simulink model "quadcopterModel"  (R2018b)
settings: Solver=ode1  StartTime=0.0  StopTime=param.tfinal  FixedStep=param.dt  RelTol=1e-3
values from neighbouring files (symbols this model uses):
  acc_acom = [1 om_com]    [quadSimRunMain.m]
  acc_bcom = [0 om_com]    [quadSimRunMain.m]
  agyro = 1    [quadSimRunMain.m]
  bgyro = 1    [quadSimRunMain.m]
  gainAcc = 1    [quadSimRunMain.m]
  gainGyro = 1    [quadSimRunMain.m]
  gainPsi = 1    [quadSimRunMain.m]
  gainWind = 1    [quadSimRunMain.m]
  gyro_acom = [1 om_com]    [quadSimRunMain.m]
  gyro_bcom = [1 0]    [quadSimRunMain.m]
  Kdphi = 0.0478*1    (= 0.0478)    [quadSimRunMain.m]
  Kdpsi = 0.067644*1    (= 0.067644)    [quadSimRunMain.m]
  Kdtheta = 0.0478*1    (= 0.0478)    [quadSimRunMain.m]
  Kdx = 15    [quadSimRunMain.m]
  Kdy = 15    [quadSimRunMain.m]
  Kdz = 5.5    [quadSimRunMain.m]
  Kiphi = 0.0098*0    (= 0)    [quadSimRunMain.m]
  Kipsi = 0.045028*.0    (= 0)    [quadSimRunMain.m]
  Kitheta = 0.0098*0    (= 0)    [quadSimRunMain.m]
  Kix = 1    [quadSimRunMain.m]
  Kiy = 1    [quadSimRunMain.m]
  Kiz = 1.5    [quadSimRunMain.m]
  Kpphi = 0.0439*1    (= 0.0439)    [quadSimRunMain.m]
  Kppsi = 0.11038*1    (= 0.11038)    [quadSimRunMain.m]
  Kptheta = 0.0439*1    (= 0.0439)    [quadSimRunMain.m]
  Kpx = 5    [quadSimRunMain.m]
  Kpy = 5    [quadSimRunMain.m]
  Kpz = 3.5    [quadSimRunMain.m]
  Nphi = 1/Tfphi    (= 162.638649449)    [quadSimRunMain.m]
  Npsi = 1/Tfpsi    (= 159.182438993)    [quadSimRunMain.m]
  Ntheta = 1/Tftheta    (= 162.638649449)    [quadSimRunMain.m]
  Nx = 1/0.002099    (= 476.417341591)    [quadSimRunMain.m]
  Ny = 1/0.002099    (= 476.417341591)    [quadSimRunMain.m]
  Nz = 1/0.002099    (= 476.417341591)    [quadSimRunMain.m]
  param = quadparam    [quadDyn.m]    (also in quadDynSimple.m; quadSimRunMain.m; quadcomputeFandT.m; quadcomputeMotorSpeed.m)
  pathSelect = 1    [quadSimRunMain.m]
  windConstant = 1    [quadSimRunMain.m]
  windVarying = 1    [quadSimRunMain.m]
undefined symbols (not defined in the file or in its folder): aHu, aHv, aHw, bHu, bHv, bHw, DiscIntNeverNeededParam
libraries: simulink x7, sharedutil x4
(part 1 of 2)
settings Model: Creator=duho46  LastModifiedBy=duho46

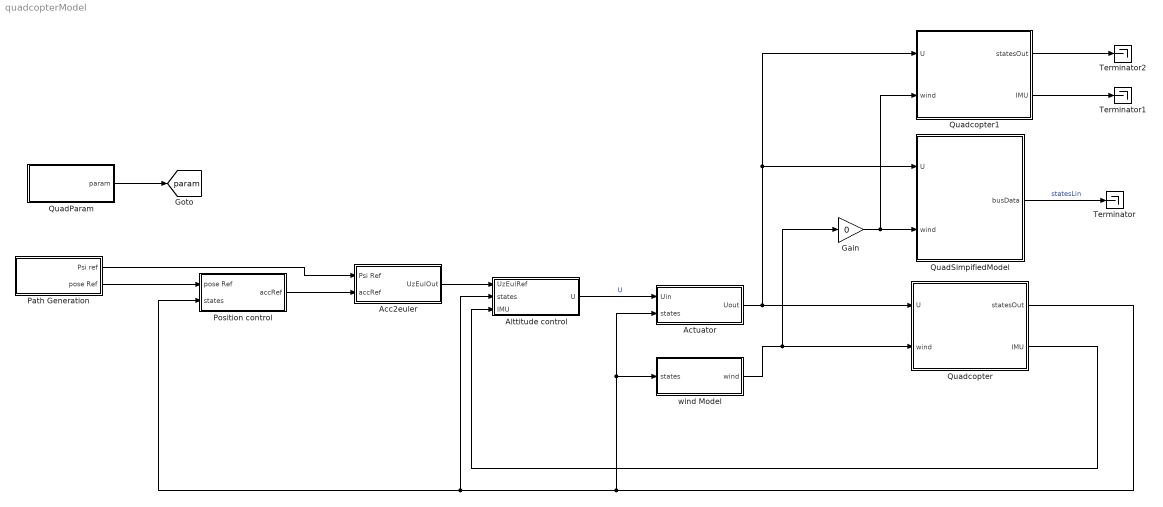
== system quadcopterModel ==
  Acc2euler : Subsystem
  Actuator : Subsystem
  Alttitude control : Subsystem
  Gain : Gain  Gain=0
  Path Generation : Subsystem
  Position control : Subsystem
  QuadParam : Subsystem
  QuadSimpifiedModel : Subsystem
      mask Display: image('C:\Users\duho46\Pictures\DJI Mavic Pro.jpg');
  Quadcopter : Subsystem
  Quadcopter1 : Subsystem
  Terminator : Terminator
  Terminator1 : Terminator
  Terminator2 : Terminator
  wind Model : Subsystem
  tag scope: param=global
  wires:
  Position control/1(accRef) -> Acc2euler/2(accRef)
  Acc2euler/1(UzEulOut) -> Alttitude control/1(UzEulRef)
  Alttitude control/1(U) -> Actuator/1(Uin)  "U"
  Actuator/1(Uout) -> Quadcopter1/1(U), QuadSimpifiedModel/1(U), Quadcopter/1(U)
  Path Generation/2(pose Ref) -> Position control/1(pose Ref)
  Quadcopter/1(statesOut) -> wind Model/1(states), Actuator/2(states), Alttitude control/2(states), Position control/2(states)
  Path Generation/1(Psi ref) -> Acc2euler/1(Psi Ref)
  wind Model/1(wind) -> Gain/1, Quadcopter/2(wind)
  QuadSimpifiedModel/1(busData) -> Terminator/1  "statesLin"
  Quadcopter/2(IMU) -> Alttitude control/3(IMU)
  Gain/1 -> Quadcopter1/2(wind), QuadSimpifiedModel/2(wind)
  QuadParam/1(param) -> [param]
  Quadcopter1/1(statesOut) -> Terminator2/1
  Quadcopter1/2(IMU) -> Terminator1/1

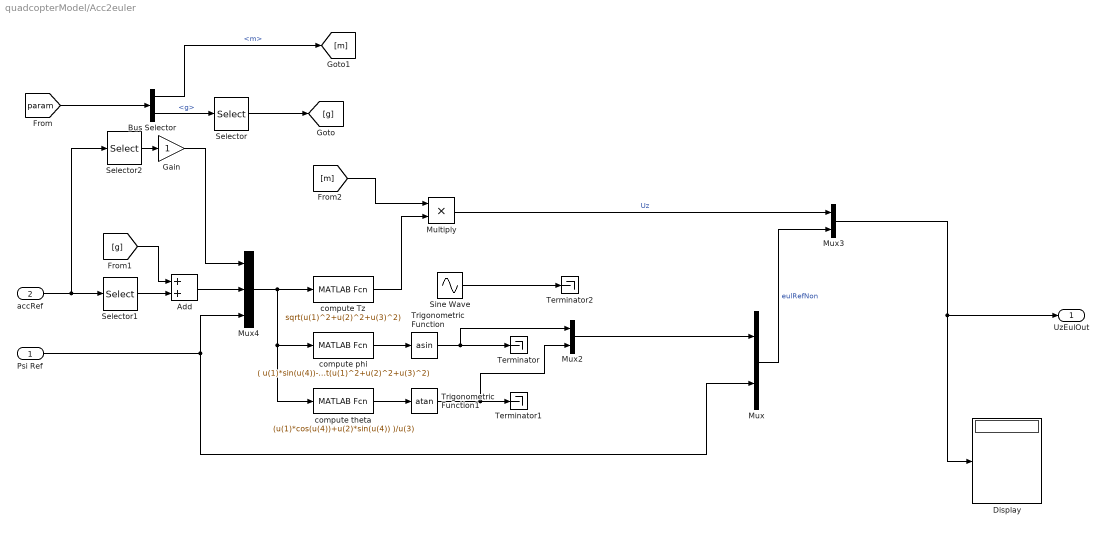
== system quadcopterModel/Acc2euler ==
  Psi Ref : Inport
  accRef : Inport  Port=2
  Add : Sum
  Bus Selector : BusSelector  OutputSignals=m,g
  Display : Display
  Gain : Gain
  Multiply : Product
  Mux : Mux  Inputs=2
  Mux2 : Mux  Inputs=2
  Mux3 : Mux  Inputs=2
  Mux4 : Mux  Inputs=3
  Selector : Selector  InputPortWidth=3  IndexOptions=Index vector (dialog)  Indices=3  OutputSizes=1
  Selector1 : Selector  InputPortWidth=3  IndexOptions=Index vector (dialog)  Indices=3  OutputSizes=1
  Selector2 : Selector  InputPortWidth=3  IndexOptions=Index vector (dialog)  Indices=[1 2]  OutputSizes=1
  Sine Wave : Sin  Amplitude=0.1  Frequency=0.2  SampleTime=0
  Terminator : Terminator
  Terminator1 : Terminator
  Terminator2 : Terminator
  Trigonometric Function : Trigonometry  Operator=asin
  Trigonometric Function1 : Trigonometry  Operator=atan
  compute Tz : MATLABFcn  MATLABFcn=sqrt(u(1)^2+u(2)^2+u(3)^2)  OutputDimensions=1  Output1D=off
  compute phi : MATLABFcn  MATLABFcn=( u(1)*sin(u(4))-u(2)*cos(u(4)) )/sqrt(u(1)^2+u(2)^2+u(3)^2)  OutputDimensions=1  Output1D=off
  compute theta : MATLABFcn  MATLABFcn=(u(1)*cos(u(4))+u(2)*sin(u(4)) )/u(3)  OutputDimensions=1  Output1D=off
  UzEulOut : Outport
  wires:
  [param] -> Bus Selector/1
  Bus Selector/2 -> Selector/1  "<g>"
  Selector/1 -> [g]
  Bus Selector/1 -> [m]  "<m>"
  accRef/1 -> Selector2/1, Selector1/1
  Selector1/1 -> Add/2
  [g] -> Add/1
  Add/1 -> Mux4/2
  [m] -> Multiply/1
  Psi Ref/1 -> Mux/2, Mux4/3
  Multiply/1 -> Mux3/1  "Uz"
  Selector2/1 -> Gain/1
  Mux/1 -> Mux3/2  "eulRefNon"
  Mux4/1 -> compute theta/1, compute phi/1, compute Tz/1
  compute phi/1 -> Trigonometric Function/1
  compute theta/1 -> Trigonometric Function1/1
  Mux3/1 -> Display/1, UzEulOut/1
  Trigonometric Function/1 -> Mux2/1, Terminator/1
  Trigonometric Function1/1 -> Mux2/2, Terminator1/1
  Gain/1 -> Mux4/1
  Mux2/1 -> Mux/1
  Sine Wave/1 -> Terminator2/1
  compute Tz/1 -> Multiply/2

== system quadcopterModel/Actuator ==
  Uin : Inport
  states : Inport  Port=2
  Bus Selector : BusSelector  OutputSignals=T,invT
  Constant : Constant  Value=diag([1 1 1 1])
  Display : Display
  Display1 : Display
  Multiply : Product  Multiplication=Matrix(*)
  Multiply1 : Product  Inputs=3  Multiplication=Matrix(*)
  Mux : Mux  Inputs=2
  Saturation1 : Saturate  UpperLimit=60000  LowerLimit=0
  Scope : Scope
  Scope1 : Scope
  Terminator : Terminator
  Uout : Outport
  wires:
  Uin/1 -> Mux/2, Display/1, Multiply/2
  states/1 -> Terminator/1
  [param] -> Bus Selector/1
  Multiply/1 -> Saturation1/1  "omRotor2"
  Multiply1/1 -> Mux/1, Display1/1, Uout/1
  Constant/1 -> Multiply1/1
  Bus Selector/2 -> Multiply/1  "<invT>"
  Bus Selector/1 -> Multiply1/2  "<T>"
  Mux/1 -> Scope/1
  Saturation1/1 -> Scope1/1, Multiply1/3

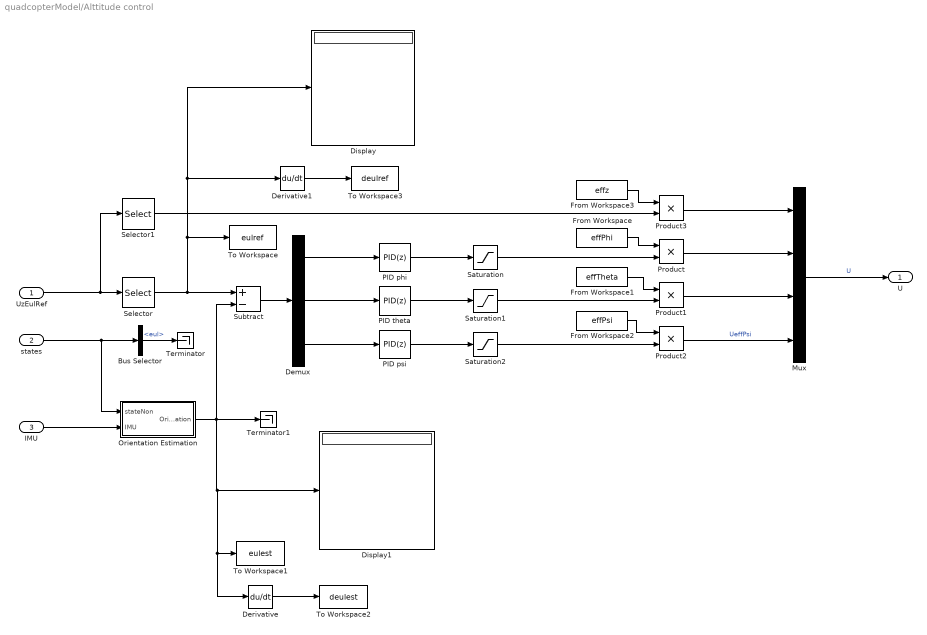
== system quadcopterModel/Alttitude control ==
  UzEulRef : Inport
  states : Inport  Port=2
  IMU : Inport  Port=3
  Bus Selector : BusSelector  OutputSignals=eul
  Demux : Demux  Outputs=3
  Derivative : Derivative
  Derivative1 : Derivative
  Display : Display
  Display1 : Display
  From Workspace : FromWorkspace  VariableName=effPhi  SampleTime=0
  From Workspace1 : FromWorkspace  VariableName=effTheta  SampleTime=0
  From Workspace2 : FromWorkspace  VariableName=effPsi  SampleTime=0
  From Workspace3 : FromWorkspace  VariableName=effz  SampleTime=0
  Mux : Mux
  Orientation Estimation : Subsystem
  PID phi : simulink/Continuous/PID Controller  Controller=PID  Form=Parallel  TimeDomain=Discrete-time  SampleTime=-1  IntegratorMethod=Forward Euler  FilterMethod=Forward Euler  ControllerParametersSource=internal  P=Kpphi  I=Kiphi*0  D=Kdphi  UseFilter=off  N=Nphi  TunerSelectOption=Transfer Function Based (PID Tuner App)  InitialConditionSource=internal  InitialConditionForIntegrator=0  InitialConditionForFilter=0  DifferentiatorICPrevScaledInput=0  ExternalReset=none  TrackingMode=off  Kt=1  LimitOutput=off  UpperSaturationLimit=inf  LowerSaturationLimit=-inf  LinearizeAsGain=on  AntiWindupMode=none  Kb=1  POutMin=[]  POutMax=[]  IOutMin=[]  IOutMax=[]  DOutMin=[]  DOutMax=[]  NOutMin=[]  NOutMax=[]  SumOutMin=[]  SumOutMax=[]  SaturationOutMin=[]  SaturationOutMax=[]  PParamMin=[]  PParamMax=[]  IParamMin=[]  IParamMax=[]  DParamMin=[]  DParamMax=[]  NParamMin=[]  NParamMax=[]  KbParamMin=[]  KbParamMax=[]  KtParamMin=[]  KtParamMax=[]  KbOutMin=[]  KbOutMax=[]  KtOutMin=[]  KtOutMax=[]  IntegratorOutMin=[]  IntegratorOutMax=[]  FilterOutMin=[]  FilterOutMax=[]  SumI1OutMin=[]  SumI1OutMax=[]  SumI2OutMin=[]  SumI2OutMax=[]  SumI3OutMin=[]  SumI3OutMax=[]  SumI4OutMin=[]  SumI4OutMax=[]  SumDOutMin=[]  SumDOutMax=[]  DifferentiatorOutMin=[]  DifferentiatorOutMax=[]  FilterDiffOutCoefMin=[]  FilterDiffOutCoefMax=[]  ReciprocalOutMin=[]  ReciprocalOutMax=[]  SumDenOutMin=[]  SumDenOutMax=[]  SumNumOutMin=[]  SumNumOutMax=[]  DivideOutMin=[]  DivideOutMax=[]  IntegratorContinuousStateAttributes=''  IntegratorStateMustResolveToSignalObject=off  IntegratorRTWStateStorageClass=Auto  FilterContinuousStateAttributes=''  FilterStateMustResolveToSignalObject=off  FilterRTWStateStorageClass=Auto  ParallelPVariant=InternalParameters  IdealPVariant=Disabled  IVariant=InternalParameters  DVariant=InternalParameters  IntegratorVariant=Discrete  SatVariant=Disabled  AWVariant=Passthrough  PCopyVariant=Disabled  TRVariant=Disabled  FdbkBlocksVariant=Forward  IdealPFdbkVariant=Disabled  SatFdbkVariant=Disabled  DerivativeFilterVariant=Differentiator  NVariant=Passthrough  NCopyVariant=Disabled_SignalSpec  FilterICVariant=InternalICsDifferentiator  IntegratorICVariant=InternalICs  ExternalResetVariant=Disabled  TRSumVariant=Passthrough  SumFdbkVariant=Disabled  SumVariant=Sum_PID
  PID psi : simulink/Continuous/PID Controller  Controller=PID  Form=Parallel  TimeDomain=Discrete-time  SampleTime=-1  IntegratorMethod=Forward Euler  FilterMethod=Forward Euler  ControllerParametersSource=internal  P=Kppsi  I=Kipsi  D=Kdpsi  UseFilter=off  N=Npsi  TunerSelectOption=Transfer Function Based (PID Tuner App)  InitialConditionSource=internal  InitialConditionForIntegrator=0  InitialConditionForFilter=0  DifferentiatorICPrevScaledInput=0  ExternalReset=none  TrackingMode=off  Kt=1  LimitOutput=off  UpperSaturationLimit=inf  LowerSaturationLimit=-inf  LinearizeAsGain=on  AntiWindupMode=none  Kb=1  POutMin=[]  POutMax=[]  IOutMin=[]  IOutMax=[]  DOutMin=[]  DOutMax=[]  NOutMin=[]  NOutMax=[]  SumOutMin=[]  SumOutMax=[]  SaturationOutMin=[]  SaturationOutMax=[]  PParamMin=[]  PParamMax=[]  IParamMin=[]  IParamMax=[]  DParamMin=[]  DParamMax=[]  NParamMin=[]  NParamMax=[]  KbParamMin=[]  KbParamMax=[]  KtParamMin=[]  KtParamMax=[]  KbOutMin=[]  KbOutMax=[]  KtOutMin=[]  KtOutMax=[]  IntegratorOutMin=[]  IntegratorOutMax=[]  FilterOutMin=[]  FilterOutMax=[]  SumI1OutMin=[]  SumI1OutMax=[]  SumI2OutMin=[]  SumI2OutMax=[]  SumI3OutMin=[]  SumI3OutMax=[]  SumI4OutMin=[]  SumI4OutMax=[]  SumDOutMin=[]  SumDOutMax=[]  DifferentiatorOutMin=[]  DifferentiatorOutMax=[]  FilterDiffOutCoefMin=[]  FilterDiffOutCoefMax=[]  ReciprocalOutMin=[]  ReciprocalOutMax=[]  SumDenOutMin=[]  SumDenOutMax=[]  SumNumOutMin=[]  SumNumOutMax=[]  DivideOutMin=[]  DivideOutMax=[]  IntegratorContinuousStateAttributes=''  IntegratorStateMustResolveToSignalObject=off  IntegratorRTWStateStorageClass=Auto  FilterContinuousStateAttributes=''  FilterStateMustResolveToSignalObject=off  FilterRTWStateStorageClass=Auto  ParallelPVariant=InternalParameters  IdealPVariant=Disabled  IVariant=InternalParameters  DVariant=InternalParameters  IntegratorVariant=Discrete  SatVariant=Disabled  AWVariant=Passthrough  PCopyVariant=Disabled  TRVariant=Disabled  FdbkBlocksVariant=Forward  IdealPFdbkVariant=Disabled  SatFdbkVariant=Disabled  DerivativeFilterVariant=Differentiator  NVariant=Passthrough  NCopyVariant=Disabled_SignalSpec  FilterICVariant=InternalICsDifferentiator  IntegratorICVariant=InternalICs  ExternalResetVariant=Disabled  TRSumVariant=Passthrough  SumFdbkVariant=Disabled  SumVariant=Sum_PID
  PID theta : simulink/Continuous/PID Controller  Controller=PID  Form=Parallel  TimeDomain=Discrete-time  SampleTime=-1  IntegratorMethod=Forward Euler  FilterMethod=Forward Euler  ControllerParametersSource=internal  P=Kptheta  I=Kitheta*0  D=Kdtheta  UseFilter=off  N=Ntheta  TunerSelectOption=Transfer Function Based (PID Tuner App)  InitialConditionSource=internal  InitialConditionForIntegrator=0  InitialConditionForFilter=0  DifferentiatorICPrevScaledInput=0  ExternalReset=none  TrackingMode=off  Kt=1  LimitOutput=off  UpperSaturationLimit=inf  LowerSaturationLimit=-inf  LinearizeAsGain=on  AntiWindupMode=none  Kb=1  POutMin=[]  POutMax=[]  IOutMin=[]  IOutMax=[]  DOutMin=[]  DOutMax=[]  NOutMin=[]  NOutMax=[]  SumOutMin=[]  SumOutMax=[]  SaturationOutMin=[]  SaturationOutMax=[]  PParamMin=[]  PParamMax=[]  IParamMin=[]  IParamMax=[]  DParamMin=[]  DParamMax=[]  NParamMin=[]  NParamMax=[]  KbParamMin=[]  KbParamMax=[]  KtParamMin=[]  KtParamMax=[]  KbOutMin=[]  KbOutMax=[]  KtOutMin=[]  KtOutMax=[]  IntegratorOutMin=[]  IntegratorOutMax=[]  FilterOutMin=[]  FilterOutMax=[]  SumI1OutMin=[]  SumI1OutMax=[]  SumI2OutMin=[]  SumI2OutMax=[]  SumI3OutMin=[]  SumI3OutMax=[]  SumI4OutMin=[]  SumI4OutMax=[]  SumDOutMin=[]  SumDOutMax=[]  DifferentiatorOutMin=[]  DifferentiatorOutMax=[]  FilterDiffOutCoefMin=[]  FilterDiffOutCoefMax=[]  ReciprocalOutMin=[]  ReciprocalOutMax=[]  SumDenOutMin=[]  SumDenOutMax=[]  SumNumOutMin=[]  SumNumOutMax=[]  DivideOutMin=[]  DivideOutMax=[]  IntegratorContinuousStateAttributes=''  IntegratorStateMustResolveToSignalObject=off  IntegratorRTWStateStorageClass=Auto  FilterContinuousStateAttributes=''  FilterStateMustResolveToSignalObject=off  FilterRTWStateStorageClass=Auto  ParallelPVariant=InternalParameters  IdealPVariant=Disabled  IVariant=InternalParameters  DVariant=InternalParameters  IntegratorVariant=Discrete  SatVariant=Disabled  AWVariant=Passthrough  PCopyVariant=Disabled  TRVariant=Disabled  FdbkBlocksVariant=Forward  IdealPFdbkVariant=Disabled  SatFdbkVariant=Disabled  DerivativeFilterVariant=Differentiator  NVariant=Passthrough  NCopyVariant=Disabled_SignalSpec  FilterICVariant=InternalICsDifferentiator  IntegratorICVariant=InternalICs  ExternalResetVariant=Disabled  TRSumVariant=Passthrough  SumFdbkVariant=Disabled  SumVariant=Sum_PID
  Product{,1..3} (4 alike) : Product
  Saturation : Saturate  UpperLimit=1  LowerLimit=-1
  Saturation1 : Saturate  UpperLimit=1  LowerLimit=-1
  Saturation2 : Saturate  UpperLimit=10  LowerLimit=-10
  Selector : Selector  InputPortWidth=4  IndexOptions=Index vector (dialog)  Indices=[2 3 4]  OutputSizes=1
  Selector1 : Selector  InputPortWidth=4  IndexOptions=Index vector (dialog)  Indices=1  OutputSizes=1
  Subtract : Sum  Inputs=+-
  Terminator : Terminator
  Terminator1 : Terminator
  To Workspace : ToWorkspace  VariableName=eulref  SampleTime=-1
  To Workspace1 : ToWorkspace  VariableName=eulest  SampleTime=-1
  To Workspace2 : ToWorkspace  VariableName=deulest  SampleTime=-1
  To Workspace3 : ToWorkspace  VariableName=deulref  SampleTime=-1
  U : Outport
  wires:
  states/1 -> Orientation Estimation/1(stateNon), Bus Selector/1
  UzEulRef/1 -> Selector1/1, Selector/1
  Product3/1 -> Mux/1
  From Workspace3/1 -> Product3/1
  Demux/1 -> PID phi/1
  From Workspace2/1 -> Product2/1
  Product2/1 -> Mux/4  "UeffPsi"
  Mux/1 -> U/1  "U"
  Selector1/1 -> Product3/2
  PID psi/1 -> Saturation2/1
  Product1/1 -> Mux/3
  From Workspace1/1 -> Product1/1
  Demux/3 -> PID psi/1
  PID theta/1 -> Saturation1/1
  Product/1 -> Mux/2
  PID phi/1 -> Saturation/1
  Demux/2 -> PID theta/1
  From Workspace/1 -> Product/1
  Subtract/1 -> Demux/1
  Selector/1 -> To Workspace/1, Derivative1/1, Display/1, Subtract/1
  IMU/1 -> Orientation Estimation/2(IMU)
  Bus Selector/1 -> Terminator/1  "<eul>"
  Orientation Estimation/1(Orientation) -> Subtract/2, Derivative/1, To Workspace1/1, Display1/1, Terminator1/1
  Saturation/1 -> Product/2
  Saturation1/1 -> Product1/2
  Saturation2/1 -> Product2/2
  Derivative/1 -> To Workspace2/1
  Derivative1/1 -> To Workspace3/1

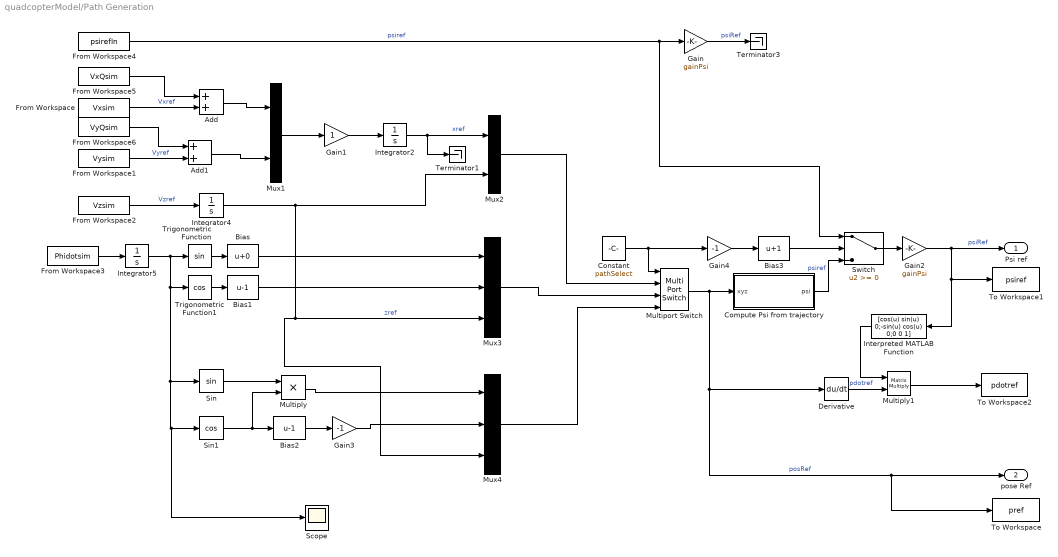
== system quadcopterModel/Path Generation ==
  Add : Sum
  Add1 : Sum
  Bias : Bias
  Bias1 : Bias  Bias=-1
  Bias2 : Bias  Bias=-1
  Bias3 : Bias  Bias=1
  Compute Psi from trajectory : Subsystem
  Constant : Constant  Value=pathSelect
  Derivative : Derivative
  From Workspace : FromWorkspace  VariableName=Vxsim  SampleTime=0
  From Workspace1 : FromWorkspace  VariableName=Vysim  SampleTime=0
  From Workspace2 : FromWorkspace  VariableName=Vzsim  SampleTime=0
  From Workspace3 : FromWorkspace  VariableName=Phidotsim  SampleTime=0
  From Workspace4 : FromWorkspace  VariableName=psirefIn  SampleTime=0
  From Workspace5 : FromWorkspace  VariableName=VxQsim  SampleTime=0
  From Workspace6 : FromWorkspace  VariableName=VyQsim  SampleTime=0
  Gain : Gain  Gain=gainPsi
  Gain1 : Gain
  Gain2 : Gain  Gain=gainPsi
  Gain3 : Gain  Gain=-1
  Gain4 : Gain  Gain=-1
  Integrator2 : Integrator
  Integrator4 : Integrator  InitialCondition=8
  Integrator5 : Integrator
  Interpreted MATLAB Function : MATLABFcn  MATLABFcn=[cos(u) sin(u) 0;-sin(u) cos(u) 0;0 0 1]  OutputDimensions=[3 3]  Output1D=off
  Multiply : Product
  Multiply1 : Product  Multiplication=Matrix(*)
  Multiport Switch : MultiPortSwitch
  Mux1 : Mux  Inputs=2
  Mux2 : Mux  Inputs=2
  Mux3 : Mux  Inputs=3
  Mux4 : Mux  Inputs=3
  Scope : Scope
  Sin : Trigonometry
  Sin1 : Trigonometry  Operator=cos
  Switch : Switch
  Terminator1 : Terminator
  Terminator3 : Terminator
  To Workspace : ToWorkspace  VariableName=pref  SampleTime=-1
  To Workspace1 : ToWorkspace  VariableName=psiref  SampleTime=-1
  To Workspace2 : ToWorkspace  VariableName=pdotref  SampleTime=-1
  Trigonometric Function : Trigonometry
  Trigonometric Function1 : Trigonometry  Operator=cos
  Psi ref : Outport
  pose Ref : Outport  Port=2
  wires:
  Mux1/1 -> Gain1/1
  From Workspace4/1 -> Switch/1, Gain/1  "psiref"
  Bias1/1 -> Mux3/2
  Bias/1 -> Mux3/1
  Trigonometric Function/1 -> Bias/1
  Trigonometric Function1/1 -> Bias1/1
  From Workspace3/1 -> Integrator5/1
  Integrator5/1 -> Trigonometric Function/1, Scope/1, Sin1/1, Sin/1, Trigonometric Function1/1
  From Workspace2/1 -> Integrator4/1  "Vzref"
  Integrator4/1 -> Mux2/2, Mux4/3, Mux3/3  "zref"
  Gain1/1 -> Integrator2/1
  Integrator2/1 -> Mux2/1, Terminator1/1  "xref"
  Sin1/1 -> Bias2/1, Multiply/2
  Sin/1 -> Multiply/1
  Multiport Switch/1 -> Compute Psi from trajectory/1(xyz), Derivative/1, To Workspace/1, pose Ref/1  "posRef"
  Gain/1 -> Terminator3/1  "psiRef"
  Bias2/1 -> Gain3/1
  Gain2/1 -> Psi ref/1, To Workspace1/1, Interpreted MATLAB Function/1  "psiRef"
  Mux2/1 -> Multiport Switch/2
  Mux3/1 -> Multiport Switch/3
  Mux4/1 -> Multiport Switch/4
  Constant/1 -> Multiport Switch/1, Gain4/1
  Multiply/1 -> Mux4/1
  Gain3/1 -> Mux4/2
  Compute Psi from trajectory/1(psi) -> Switch/3  "psiref"
  Switch/1 -> Gain2/1
  Gain4/1 -> Bias3/1
  Bias3/1 -> Switch/2
  Interpreted MATLAB Function/1 -> Multiply1/1
  Derivative/1 -> Multiply1/2  "pdotref"
  Multiply1/1 -> To Workspace2/1
  From Workspace/1 -> Add/2  "Vxref"
  From Workspace1/1 -> Add1/2  "Vyref"
  From Workspace6/1 -> Add1/1
  Add1/1 -> Mux1/2
  Add/1 -> Mux1/1
  From Workspace5/1 -> Add/1

== system quadcopterModel/Position control ==
  pose Ref : Inport
  states : Inport  Port=2
  Bus Selector : BusSelector  OutputSignals=p
  Demux : Demux  Outputs=3
  Demux1 : Demux  Outputs=3
  Mux : Mux  Inputs=3
  PID x : simulink/Continuous/PID Controller  Controller=PID  Form=Parallel  TimeDomain=Discrete-time  SampleTime=-1  IntegratorMethod=Forward Euler  FilterMethod=Forward Euler  ControllerParametersSource=internal  P=Kpx  I=Kix  D=Kdx  UseFilter=off  N=Nx  TunerSelectOption=Transfer Function Based (PID Tuner App)  InitialConditionSource=internal  InitialConditionForIntegrator=0  InitialConditionForFilter=0  DifferentiatorICPrevScaledInput=0  ExternalReset=none  TrackingMode=off  Kt=1  LimitOutput=off  UpperSaturationLimit=inf  LowerSaturationLimit=-inf  LinearizeAsGain=on  AntiWindupMode=none  Kb=1  POutMin=[]  POutMax=[]  IOutMin=[]  IOutMax=[]  DOutMin=[]  DOutMax=[]  NOutMin=[]  NOutMax=[]  SumOutMin=[]  SumOutMax=[]  SaturationOutMin=[]  SaturationOutMax=[]  PParamMin=[]  PParamMax=[]  IParamMin=[]  IParamMax=[]  DParamMin=[]  DParamMax=[]  NParamMin=[]  NParamMax=[]  KbParamMin=[]  KbParamMax=[]  KtParamMin=[]  KtParamMax=[]  KbOutMin=[]  KbOutMax=[]  KtOutMin=[]  KtOutMax=[]  IntegratorOutMin=[]  IntegratorOutMax=[]  FilterOutMin=[]  FilterOutMax=[]  SumI1OutMin=[]  SumI1OutMax=[]  SumI2OutMin=[]  SumI2OutMax=[]  SumI3OutMin=[]  SumI3OutMax=[]  SumI4OutMin=[]  SumI4OutMax=[]  SumDOutMin=[]  SumDOutMax=[]  DifferentiatorOutMin=[]  DifferentiatorOutMax=[]  FilterDiffOutCoefMin=[]  FilterDiffOutCoefMax=[]  ReciprocalOutMin=[]  ReciprocalOutMax=[]  SumDenOutMin=[]  SumDenOutMax=[]  SumNumOutMin=[]  SumNumOutMax=[]  DivideOutMin=[]  DivideOutMax=[]  IntegratorContinuousStateAttributes=''  IntegratorStateMustResolveToSignalObject=off  IntegratorRTWStateStorageClass=Auto  FilterContinuousStateAttributes=''  FilterStateMustResolveToSignalObject=off  FilterRTWStateStorageClass=Auto  ParallelPVariant=InternalParameters  IdealPVariant=Disabled  IVariant=InternalParameters  DVariant=InternalParameters  IntegratorVariant=Discrete  SatVariant=Disabled  AWVariant=Passthrough  PCopyVariant=Disabled  TRVariant=Disabled  FdbkBlocksVariant=Forward  IdealPFdbkVariant=Disabled  SatFdbkVariant=Disabled  DerivativeFilterVariant=Differentiator  NVariant=Passthrough  NCopyVariant=Disabled_SignalSpec  FilterICVariant=InternalICsDifferentiator  IntegratorICVariant=InternalICs  ExternalResetVariant=Disabled  TRSumVariant=Passthrough  SumFdbkVariant=Disabled  SumVariant=Sum_PID
  PID y : simulink/Continuous/PID Controller  Controller=PID  Form=Parallel  TimeDomain=Discrete-time  SampleTime=-1  IntegratorMethod=Forward Euler  FilterMethod=Forward Euler  ControllerParametersSource=internal  P=Kpy  I=Kiy  D=Kdy  UseFilter=off  N=Ny  TunerSelectOption=Transfer Function Based (PID Tuner App)  InitialConditionSource=internal  InitialConditionForIntegrator=0  InitialConditionForFilter=0  DifferentiatorICPrevScaledInput=0  ExternalReset=none  TrackingMode=off  Kt=1  LimitOutput=off  UpperSaturationLimit=inf  LowerSaturationLimit=-inf  LinearizeAsGain=on  AntiWindupMode=none  Kb=1  POutMin=[]  POutMax=[]  IOutMin=[]  IOutMax=[]  DOutMin=[]  DOutMax=[]  NOutMin=[]  NOutMax=[]  SumOutMin=[]  SumOutMax=[]  SaturationOutMin=[]  SaturationOutMax=[]  PParamMin=[]  PParamMax=[]  IParamMin=[]  IParamMax=[]  DParamMin=[]  DParamMax=[]  NParamMin=[]  NParamMax=[]  KbParamMin=[]  KbParamMax=[]  KtParamMin=[]  KtParamMax=[]  KbOutMin=[]  KbOutMax=[]  KtOutMin=[]  KtOutMax=[]  IntegratorOutMin=[]  IntegratorOutMax=[]  FilterOutMin=[]  FilterOutMax=[]  SumI1OutMin=[]  SumI1OutMax=[]  SumI2OutMin=[]  SumI2OutMax=[]  SumI3OutMin=[]  SumI3OutMax=[]  SumI4OutMin=[]  SumI4OutMax=[]  SumDOutMin=[]  SumDOutMax=[]  DifferentiatorOutMin=[]  DifferentiatorOutMax=[]  FilterDiffOutCoefMin=[]  FilterDiffOutCoefMax=[]  ReciprocalOutMin=[]  ReciprocalOutMax=[]  SumDenOutMin=[]  SumDenOutMax=[]  SumNumOutMin=[]  SumNumOutMax=[]  DivideOutMin=[]  DivideOutMax=[]  IntegratorContinuousStateAttributes=''  IntegratorStateMustResolveToSignalObject=off  IntegratorRTWStateStorageClass=Auto  FilterContinuousStateAttributes=''  FilterStateMustResolveToSignalObject=off  FilterRTWStateStorageClass=Auto  ParallelPVariant=InternalParameters  IdealPVariant=Disabled  IVariant=InternalParameters  DVariant=InternalParameters  IntegratorVariant=Discrete  SatVariant=Disabled  AWVariant=Passthrough  PCopyVariant=Disabled  TRVariant=Disabled  FdbkBlocksVariant=Forward  IdealPFdbkVariant=Disabled  SatFdbkVariant=Disabled  DerivativeFilterVariant=Differentiator  NVariant=Passthrough  NCopyVariant=Disabled_SignalSpec  FilterICVariant=InternalICsDifferentiator  IntegratorICVariant=InternalICs  ExternalResetVariant=Disabled  TRSumVariant=Passthrough  SumFdbkVariant=Disabled  SumVariant=Sum_PID
  PID z : simulink/Continuous/PID Controller  Controller=PID  Form=Parallel  TimeDomain=Discrete-time  SampleTime=-1  IntegratorMethod=Forward Euler  FilterMethod=Forward Euler  ControllerParametersSource=internal  P=Kpz  I=Kiz  D=Kdz  UseFilter=off  N=Nz  TunerSelectOption=Transfer Function Based (PID Tuner App)  InitialConditionSource=internal  InitialConditionForIntegrator=0  InitialConditionForFilter=0  DifferentiatorICPrevScaledInput=0  ExternalReset=none  TrackingMode=off  Kt=1  LimitOutput=off  UpperSaturationLimit=inf  LowerSaturationLimit=-inf  LinearizeAsGain=on  AntiWindupMode=none  Kb=1  POutMin=[]  POutMax=[]  IOutMin=[]  IOutMax=[]  DOutMin=[]  DOutMax=[]  NOutMin=[]  NOutMax=[]  SumOutMin=[]  SumOutMax=[]  SaturationOutMin=[]  SaturationOutMax=[]  PParamMin=[]  PParamMax=[]  IParamMin=[]  IParamMax=[]  DParamMin=[]  DParamMax=[]  NParamMin=[]  NParamMax=[]  KbParamMin=[]  KbParamMax=[]  KtParamMin=[]  KtParamMax=[]  KbOutMin=[]  KbOutMax=[]  KtOutMin=[]  KtOutMax=[]  IntegratorOutMin=[]  IntegratorOutMax=[]  FilterOutMin=[]  FilterOutMax=[]  SumI1OutMin=[]  SumI1OutMax=[]  SumI2OutMin=[]  SumI2OutMax=[]  SumI3OutMin=[]  SumI3OutMax=[]  SumI4OutMin=[]  SumI4OutMax=[]  SumDOutMin=[]  SumDOutMax=[]  DifferentiatorOutMin=[]  DifferentiatorOutMax=[]  FilterDiffOutCoefMin=[]  FilterDiffOutCoefMax=[]  ReciprocalOutMin=[]  ReciprocalOutMax=[]  SumDenOutMin=[]  SumDenOutMax=[]  SumNumOutMin=[]  SumNumOutMax=[]  DivideOutMin=[]  DivideOutMax=[]  IntegratorContinuousStateAttributes=''  IntegratorStateMustResolveToSignalObject=off  IntegratorRTWStateStorageClass=Auto  FilterContinuousStateAttributes=''  FilterStateMustResolveToSignalObject=off  FilterRTWStateStorageClass=Auto  ParallelPVariant=InternalParameters  IdealPVariant=Disabled  IVariant=InternalParameters  DVariant=InternalParameters  IntegratorVariant=Discrete  SatVariant=Disabled  AWVariant=Passthrough  PCopyVariant=Disabled  TRVariant=Disabled  FdbkBlocksVariant=Forward  IdealPFdbkVariant=Disabled  SatFdbkVariant=Disabled  DerivativeFilterVariant=Differentiator  NVariant=Passthrough  NCopyVariant=Disabled_SignalSpec  FilterICVariant=InternalICsDifferentiator  IntegratorICVariant=InternalICs  ExternalResetVariant=Disabled  TRSumVariant=Passthrough  SumFdbkVariant=Disabled  SumVariant=Sum_PID
  Scope : Scope
  Scope1 : Scope
  Sum : Sum  Inputs=|+-
  Terminator : Terminator
  To Workspace : ToWorkspace  VariableName=accRef  SampleTime=-1
  accRef : Outport
  wires:
  Sum/1 -> Demux1/1, Demux/1
  Demux/2 -> PID y/1
  Demux/1 -> PID x/1
  pose Ref/1 -> Sum/1
  Mux/1 -> To Workspace/1, accRef/1  "accRef"
  PID z/1 -> Mux/3
  PID y/1 -> Mux/2
  PID x/1 -> Mux/1
  Demux/3 -> PID z/1
  states/1 -> Bus Selector/1
  Bus Selector/1 -> Sum/2  "<p>"
  Demux1/1 -> Scope/1
  Demux1/2 -> Scope1/1
  Demux1/3 -> Terminator/1

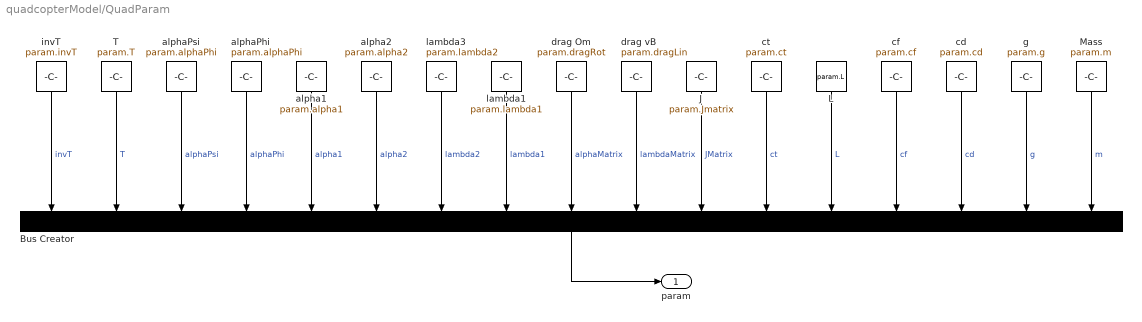
== system quadcopterModel/QuadParam ==
  Bus Creator : BusCreator  Inputs=17
  J : Constant  Value=param.Jmatrix  VectorParams1D=off  OutDataTypeStr=double  SampleTime=-1
  L : Constant  Value=param.L
  Mass : Constant  Value=param.m
  T : Constant  Value=param.T
  "alpha1 " : Constant  Value=param.alpha1
  alpha2 : Constant  Value=param.alpha2
  alphaPhi : Constant  Value=param.alphaPhi
  alphaPsi : Constant  Value=param.alphaPhi
  cd : Constant  Value=param.cd
  cf : Constant  Value=param.cf
  ct : Constant  Value=param.ct
  drag Om : Constant  Value=param.dragRot  VectorParams1D=off
  drag vB : Constant  Value=param.dragLin  VectorParams1D=off
  g : Constant  Value=param.g
  invT : Constant  Value=param.invT
  lambda1 : Constant  Value=param.lambda1
  lambda3 : Constant  Value=param.lambda2
  param : Outport
  wires:
  invT/1 -> Bus Creator/1  "invT"
  T/1 -> Bus Creator/2  "T"
  alphaPsi/1 -> Bus Creator/3  "alphaPsi"
  alphaPhi/1 -> Bus Creator/4  "alphaPhi"
  "alpha1 "/1 -> Bus Creator/5  "alpha1"
  alpha2/1 -> Bus Creator/6  "alpha2"
  lambda3/1 -> Bus Creator/7  "lambda2"
  lambda1/1 -> Bus Creator/8  "lambda1"
  drag Om/1 -> Bus Creator/9  "alphaMatrix"
  drag vB/1 -> Bus Creator/10  "lambdaMatrix"
  J/1 -> Bus Creator/11  "JMatrix"
  ct/1 -> Bus Creator/12  "ct"
  L/1 -> Bus Creator/13  "L"
  cf/1 -> Bus Creator/14  "cf"
  cd/1 -> Bus Creator/15  "cd"
  g/1 -> Bus Creator/16  "g"
  Mass/1 -> Bus Creator/17  "m"
  Bus Creator/1 -> param/1

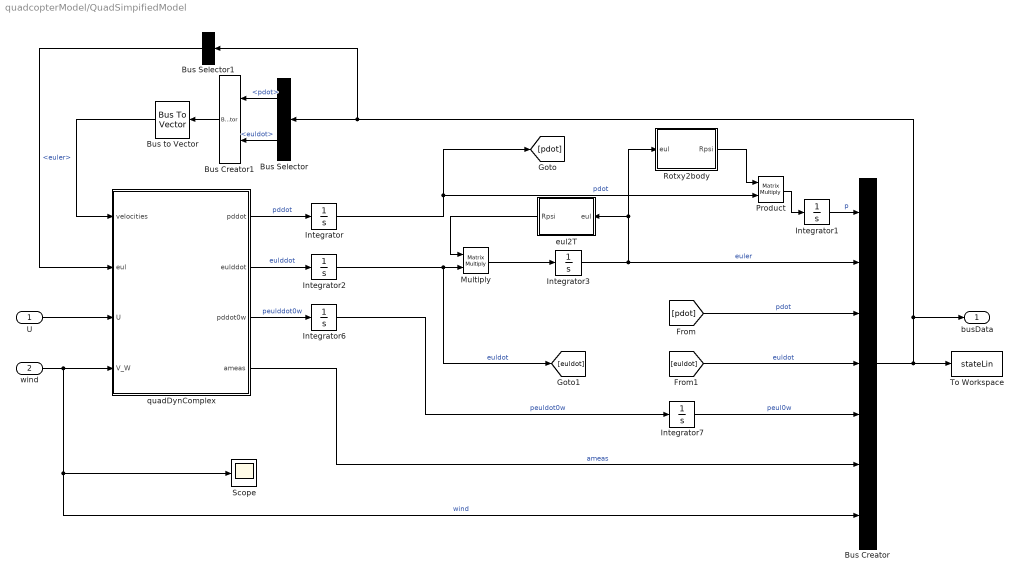
== system quadcopterModel/QuadSimpifiedModel ==
  U : Inport
  wind : Inport  Port=2
  Bus Creator : BusCreator  Inputs=7
  Bus Creator1 : BusCreator  Inputs=2
  Bus Selector : BusSelector  OutputSignals=pdot,euldot
  Bus Selector1 : BusSelector  OutputSignals=euler
  Bus to Vector : BusToVector
  Integrator : Integrator  InitialCondition=[0 0 0]
  Integrator1 : Integrator  InitialCondition=[0 0 8]
  Integrator2 : Integrator  InitialCondition=[0 0 0]
  Integrator3 : Integrator  InitialCondition=[0 0 0]
  Integrator6 : Integrator  InitialCondition=[0 0 0 0 0 0]
  Integrator7 : Integrator  InitialCondition=[0 0 0 0 0 0]
  Multiply : Product  Multiplication=Matrix(*)
  Product : Product  Multiplication=Matrix(*)
  Rotxy2body : MATLAB Function  TreatAsAtomicUnit=on
  Scope : Scope
  To Workspace : ToWorkspace  VariableName=stateLin  SampleTime=-1
  eul2T : MATLAB Function  TreatAsAtomicUnit=on
  quadDynComplex : MATLAB Function  TreatAsAtomicUnit=on
  busData : Outport
  wires:
  wind/1 -> Scope/1, Bus Creator/7, quadDynComplex/4(V_W)  "wind"
  Integrator6/1 -> Integrator7/1  "peuldot0w"
  quadDynComplex/3(pddot0w) -> Integrator6/1  "peulddot0w"
  U/1 -> quadDynComplex/3(U)
  Integrator1/1 -> Bus Creator/1  "p"
  Integrator7/1 -> Bus Creator/5  "peul0w"
  Bus Creator/1 -> Bus Selector1/1, Bus Selector/1, busData/1, To Workspace/1
  Bus Selector/1 -> Bus Creator1/1  "<pdot>"
  Bus Selector/2 -> Bus Creator1/2  "<euldot>"
  Bus Creator1/1 -> Bus to Vector/1
  Bus to Vector/1 -> quadDynComplex/1(velocities)
  Bus Selector1/1 -> quadDynComplex/2(eul)  "<euler>"
  [pdot] -> Bus Creator/3  "pdot"
  Integrator3/1 -> eul2T/1(eul), Rotxy2body/1(eul), Bus Creator/2  "euler"
  quadDynComplex/1(pddot) -> Integrator/1  "pddot"
  quadDynComplex/2(eulddot) -> Integrator2/1  "eulddot"
  Integrator/1 -> [pdot], Product/2  "pdot"
  [euldot] -> Bus Creator/4  "euldot"
  quadDynComplex/4(ameas) -> Bus Creator/6  "ameas"
  Rotxy2body/1(Rpsi) -> Product/1
  Product/1 -> Integrator1/1
  Multiply/1 -> Integrator3/1
  eul2T/1(Rpsi) -> Multiply/1
  Integrator2/1 -> [euldot], Multiply/2  "euldot"

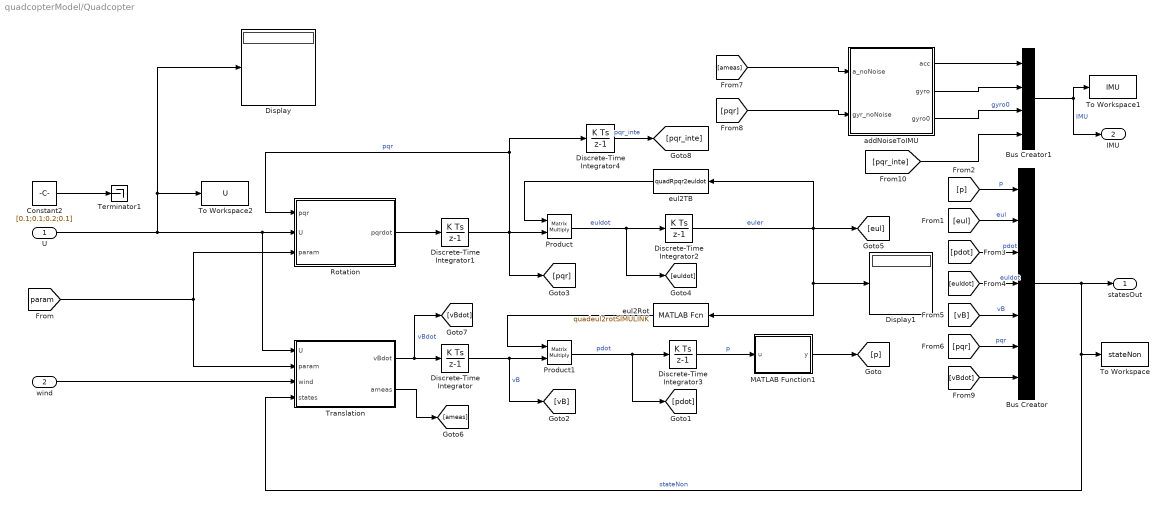
== system quadcopterModel/Quadcopter ==
  U : Inport
  wind : Inport  Port=2
  Bus Creator : BusCreator  Inputs=7
  Bus Creator1 : BusCreator  Inputs=4
  Constant2 : Constant  Value=[0.1;0.1;0.2;0.1]  OutDataTypeStr=double  SampleTime=-1
  Discrete-Time Integrator{,1..2,4} (4 alike) : DiscreteIntegrator  SampleTime=-1  ICPrevOutput=DiscIntNeverNeededParam  ICPrevScaledInput=DiscIntNeverNeededParam
  Discrete-Time Integrator3 : DiscreteIntegrator  InitialCondition=[0 0 8]  SampleTime=-1  ICPrevOutput=DiscIntNeverNeededParam  ICPrevScaledInput=DiscIntNeverNeededParam
  Display : Display
  Display1 : Display
  MATLAB Function1 : MATLAB Function  TreatAsAtomicUnit=on
  Product : Product  Multiplication=Matrix(*)
  Product1 : Product  Multiplication=Matrix(*)
  Rotation : Subsystem
  Terminator1 : Terminator
  To Workspace : ToWorkspace  VariableName=stateNon  SampleTime=-1
  To Workspace1 : ToWorkspace  VariableName=IMU  SampleTime=-1
  To Workspace2 : ToWorkspace  VariableName=U  SampleTime=-1
  Translation : Subsystem
  addNoiseToIMU : Subsystem
  eul2Rot : MATLABFcn  MATLABFcn=quadeul2rotSIMULINK  Output1D=off
  eul2TB : MATLABFcn  MATLABFcn=quadRpqr2euldot  Output1D=off
  statesOut : Outport
  IMU : Outport  Port=2
  wires:
  Discrete-Time Integrator2/1 -> [eul], eul2TB/1, eul2Rot/1, Display1/1  "euler"
  Product/1 -> Discrete-Time Integrator2/1, [euldot]  "euldot"
  eul2TB/1 -> Product/1
  Discrete-Time Integrator/1 -> Product1/2, [vB]  "vB"
  Product1/1 -> Discrete-Time Integrator3/1, [pdot]  "pdot"
  eul2Rot/1 -> Product1/1
  Discrete-Time Integrator3/1 -> MATLAB Function1/1(u)  "p"
  Bus Creator/1 -> Translation/4(states), To Workspace/1, statesOut/1  "stateNon"
  [p] -> Bus Creator/1  "p"
  [eul] -> Bus Creator/2  "eul"
  [pdot] -> Bus Creator/3  "pdot"
  [euldot] -> Bus Creator/4  "euldot"
  [vB] -> Bus Creator/5  "vB"
  [pqr] -> Bus Creator/6  "pqr"
  [param] -> Translation/2(param), Rotation/3(param)
  Discrete-Time Integrator1/1 -> Discrete-Time Integrator4/1, Rotation/1(pqr), [pqr], Product/2  "pqr"
  Rotation/1(pqrdot) -> Discrete-Time Integrator1/1
  Translation/1(vBdot) -> Discrete-Time Integrator/1, [vBdot]  "vBdot"
  U/1 -> To Workspace2/1, Display/1, Translation/1(U), Rotation/2(U)
  Constant2/1 -> Terminator1/1
  wind/1 -> Translation/3(wind)
  Translation/2(ameas) -> [ameas]
  Bus Creator1/1 -> To Workspace1/1, IMU/1  "IMU"
  [ameas] -> addNoiseToIMU/1(a_noNoise)
  [pqr] -> addNoiseToIMU/2(gyr_noNoise)
  addNoiseToIMU/1(acc) -> Bus Creator1/1
  addNoiseToIMU/2(gyro) -> Bus Creator1/2
  [vBdot] -> Bus Creator/7
  MATLAB Function1/1(y) -> [p]
  Discrete-Time Integrator4/1 -> [pqr_inte]  "pqr_inte"
  addNoiseToIMU/3(gyro0) -> Bus Creator1/3  "gyro0"
  [pqr_inte] -> Bus Creator1/4

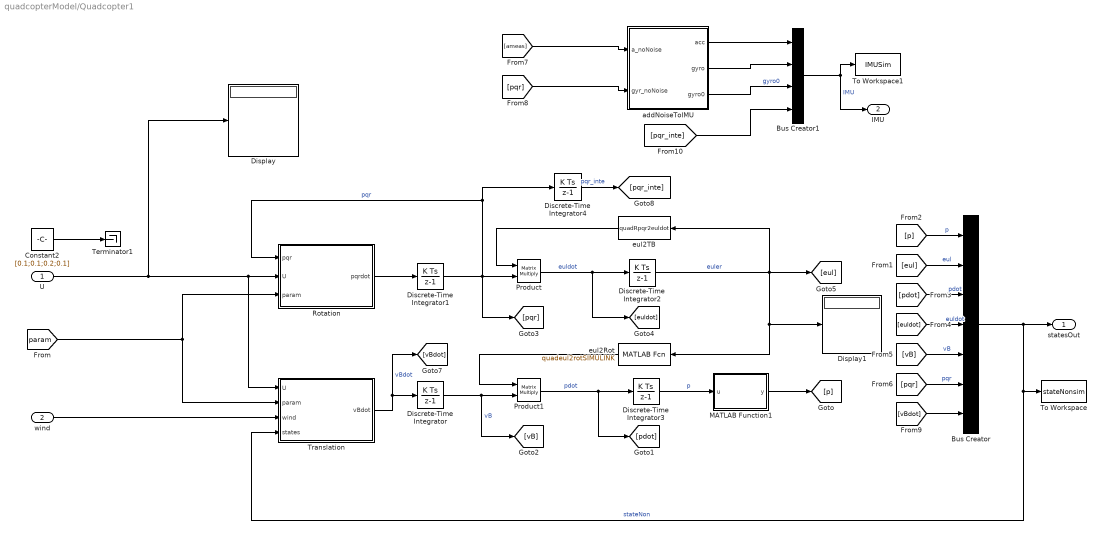
== system quadcopterModel/Quadcopter1 ==
  U : Inport
  wind : Inport  Port=2
  Bus Creator : BusCreator  Inputs=7
  Bus Creator1 : BusCreator  Inputs=4
  Constant2 : Constant  Value=[0.1;0.1;0.2;0.1]  OutDataTypeStr=double  SampleTime=-1
  Discrete-Time Integrator : DiscreteIntegrator  SampleTime=-1  ICPrevOutput=DiscIntNeverNeededParam  ICPrevScaledInput=DiscIntNeverNeededParam
  Discrete-Time Integrator1 : DiscreteIntegrator  SampleTime=-1  ICPrevOutput=DiscIntNeverNeededParam  ICPrevScaledInput=DiscIntNeverNeededParam
  Discrete-Time Integrator2 : DiscreteIntegrator  InitialCondition=[0 0 0]  SampleTime=-1  ICPrevOutput=DiscIntNeverNeededParam  ICPrevScaledInput=DiscIntNeverNeededParam
  Discrete-Time Integrator3 : DiscreteIntegrator  InitialCondition=[0 0 8]  SampleTime=-1  ICPrevOutput=DiscIntNeverNeededParam  ICPrevScaledInput=DiscIntNeverNeededParam
  Discrete-Time Integrator4 : DiscreteIntegrator  SampleTime=-1  ICPrevOutput=DiscIntNeverNeededParam  ICPrevScaledInput=DiscIntNeverNeededParam
  Display : Display
  Display1 : Display
  MATLAB Function1 : MATLAB Function  TreatAsAtomicUnit=on
  Product : Product  Multiplication=Matrix(*)
  Product1 : Product  Multiplication=Matrix(*)
  Rotation : Subsystem
  Terminator1 : Terminator
  To Workspace : ToWorkspace  VariableName=stateNonsim  SampleTime=-1
  To Workspace1 : ToWorkspace  VariableName=IMUSim  SampleTime=-1
  Translation : Subsystem
  addNoiseToIMU : Subsystem
  eul2Rot : MATLABFcn  MATLABFcn=quadeul2rotSIMULINK  Output1D=off
  eul2TB : MATLABFcn  MATLABFcn=quadRpqr2euldot  Output1D=off
  statesOut : Outport
  IMU : Outport  Port=2
  wires:
  Discrete-Time Integrator4/1 -> [pqr_inte]  "pqr_inte"
  MATLAB Function1/1(y) -> [p]
  [vBdot] -> Bus Creator/7
  wind/1 -> Translation/3(wind)
  Constant2/1 -> Terminator1/1
  U/1 -> Rotation/2(U), Translation/1(U), Display/1
  Translation/1(vBdot) -> [vBdot], Discrete-Time Integrator/1  "vBdot"
  Rotation/1(pqrdot) -> Discrete-Time Integrator1/1
  Discrete-Time Integrator1/1 -> Product/2, [pqr], Rotation/1(pqr), Discrete-Time Integrator4/1  "pqr"
  [param] -> Rotation/3(param), Translation/2(param)
  [pqr] -> Bus Creator/6  "pqr"
  [vB] -> Bus Creator/5  "vB"
  [euldot] -> Bus Creator/4  "euldot"
  [pdot] -> Bus Creator/3  "pdot"
  [eul] -> Bus Creator/2  "eul"
  [p] -> Bus Creator/1  "p"
  Bus Creator/1 -> statesOut/1, To Workspace/1, Translation/4(states)  "stateNon"
  Discrete-Time Integrator3/1 -> MATLAB Function1/1(u)  "p"
  eul2Rot/1 -> Product1/1
  Product1/1 -> [pdot], Discrete-Time Integrator3/1  "pdot"
  Discrete-Time Integrator/1 -> [vB], Product1/2  "vB"
  eul2TB/1 -> Product/1
  Product/1 -> [euldot], Discrete-Time Integrator2/1  "euldot"
  Discrete-Time Integrator2/1 -> Display1/1, eul2Rot/1, eul2TB/1, [eul]  "euler"
  [pqr_inte] -> Bus Creator1/4
  addNoiseToIMU/3(gyro0) -> Bus Creator1/3  "gyro0"
  addNoiseToIMU/2(gyro) -> Bus Creator1/2
  Bus Creator1/1 -> To Workspace1/1, IMU/1  "IMU"
  [pqr] -> addNoiseToIMU/2(gyr_noNoise)
  addNoiseToIMU/1(acc) -> Bus Creator1/1
  [ameas] -> addNoiseToIMU/1(a_noNoise)

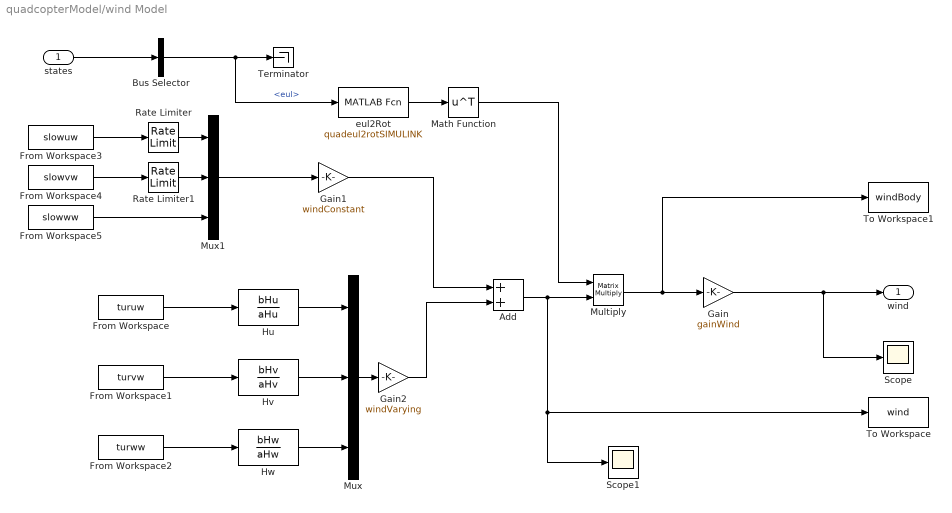
== system quadcopterModel/wind Model ==
  states : Inport
  Add : Sum
  Bus Selector : BusSelector  OutputSignals=eul
  From Workspace : FromWorkspace  VariableName=turuw  SampleTime=0
  From Workspace1 : FromWorkspace  VariableName=turvw  SampleTime=0
  From Workspace2 : FromWorkspace  VariableName=turww  SampleTime=0
  From Workspace3 : FromWorkspace  VariableName=slowuw  SampleTime=0
  From Workspace4 : FromWorkspace  VariableName=slowvw  SampleTime=0
  From Workspace5 : FromWorkspace  VariableName=slowww  SampleTime=0
  Gain : Gain  Gain=gainWind
  Gain1 : Gain  Gain=windConstant
  Gain2 : Gain  Gain=windVarying
  Hu : TransferFcn  Numerator=bHu  Denominator=aHu
  Hv : TransferFcn  Numerator=bHv  Denominator=aHv
  Hw : TransferFcn  Numerator=bHw  Denominator=aHw
  Math Function : Math  Operator=transpose  SaturateOnIntegerOverflow=on
  Multiply : Product  Multiplication=Matrix(*)
  Mux : Mux  Inputs=3
  Mux1 : Mux  Inputs=3
  Rate Limiter : RateLimiter  SampleTimeMode=inherited
  Rate Limiter1 : RateLimiter  SampleTimeMode=inherited
  Scope : Scope
  Scope1 : Scope
  Terminator : Terminator
  To Workspace : ToWorkspace  VariableName=wind  SampleTime=-1
  To Workspace1 : ToWorkspace  VariableName=windBody  SampleTime=-1
  eul2Rot : MATLABFcn  MATLABFcn=quadeul2rotSIMULINK  Output1D=off
  wind : Outport
  wires:
  states/1 -> Bus Selector/1
  Bus Selector/1 -> eul2Rot/1, Terminator/1  "<eul>"
  Gain/1 -> Scope/1, wind/1
  Hu/1 -> Mux/1
  Hv/1 -> Mux/2
  Hw/1 -> Mux/3
  From Workspace/1 -> Hu/1
  From Workspace1/1 -> Hv/1
  From Workspace2/1 -> Hw/1
  eul2Rot/1 -> Math Function/1
  From Workspace3/1 -> Rate Limiter/1
  From Workspace4/1 -> Rate Limiter1/1
  From Workspace5/1 -> Mux1/3
  Mux1/1 -> Gain1/1
  Rate Limiter/1 -> Mux1/1
  Rate Limiter1/1 -> Mux1/2
  Mux/1 -> Gain2/1
  Gain1/1 -> Add/1
  Add/1 -> To Workspace/1, Scope1/1, Multiply/2
  Multiply/1 -> To Workspace1/1, Gain/1
  Math Function/1 -> Multiply/1
  Gain2/1 -> Add/2

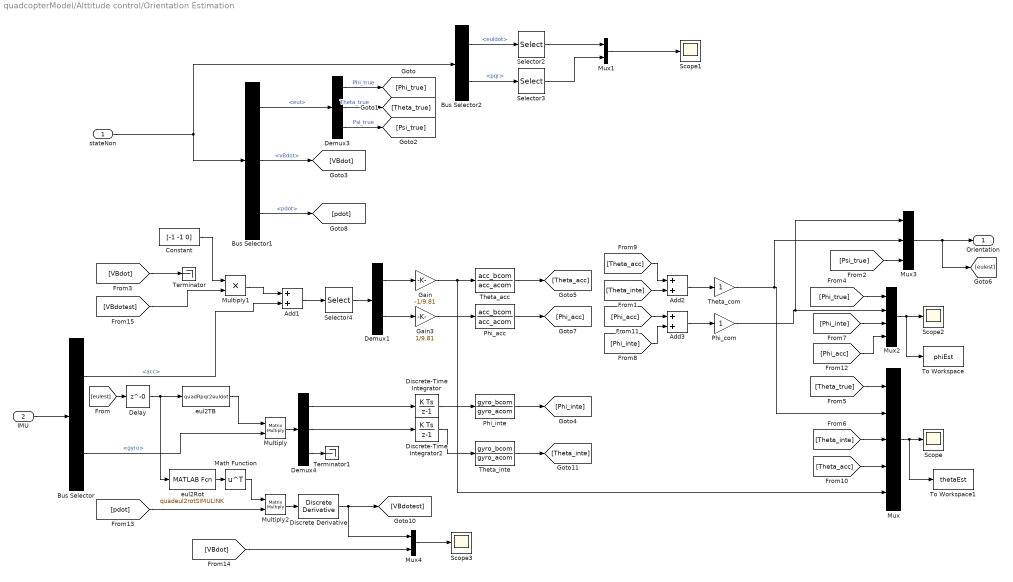
== system quadcopterModel/Alttitude control/Orientation Estimation ==
  stateNon : Inport
  IMU : Inport  Port=2
  Add1 : Sum
  Add2 : Sum
  Add3 : Sum
  Bus Selector : BusSelector  OutputSignals=acc,gyro
  Bus Selector1 : BusSelector  OutputSignals=eul,vBdot,pdot
  Bus Selector2 : BusSelector  OutputSignals=euldot,pqr
  Constant : Constant  Value=[-1 -1 0]
  Delay : Delay  DelayLength=0
  Demux1 : Demux  Outputs=2
  Demux3 : Demux  Outputs=3
  Demux4 : Demux  Outputs=3
  Discrete Derivative : simulink/Discrete/Discrete Derivative  gainval=1.0  ICPrevScaledInput=0.0  OutMin=[]  OutMax=[]  OutDataType=fixdt(1, 16)  OutScaling=2^-10  DoSatur=off
  Discrete-Time Integrator : DiscreteIntegrator  SampleTime=-1  ICPrevOutput=DiscIntNeverNeededParam  ICPrevScaledInput=DiscIntNeverNeededParam
  Discrete-Time Integrator2 : DiscreteIntegrator  SampleTime=-1  ICPrevOutput=DiscIntNeverNeededParam  ICPrevScaledInput=DiscIntNeverNeededParam
  Gain : Gain  Gain=-1/9.81
  Gain3 : Gain  Gain=1/9.81
  Math Function : Math  Operator=transpose  SaturateOnIntegerOverflow=on
  Multiply : Product  Multiplication=Matrix(*)
  Multiply1 : Product
  Multiply2 : Product  Multiplication=Matrix(*)
  Mux : Mux  Inputs=5
  Mux1 : Mux  Inputs=2
  Mux2 : Mux
  Mux3 : Mux  Inputs=3
  Mux4 : Mux  Inputs=2
  Phi_acc : TransferFcn  Numerator=acc_bcom  Denominator=acc_acom
  Phi_com : Gain
  Phi_inte : TransferFcn  Numerator=gyro_bcom  Denominator=gyro_acom
  Scope{,1..3} (4 alike) : Scope
  Selector2 : Selector  InputPortWidth=3  IndexOptions=Index vector (dialog)  Indices=[1 2]  OutputSizes=1
  Selector3 : Selector  InputPortWidth=3  IndexOptions=Index vector (dialog)  Indices=[1 2]  OutputSizes=1
  Selector4 : Selector  InputPortWidth=3  IndexOptions=Index vector (dialog)  Indices=[1 2]  OutputSizes=1
  Terminator : Terminator
  Terminator1 : Terminator
  Theta_acc : TransferFcn  Numerator=acc_bcom  Denominator=acc_acom
  Theta_com : Gain
  Theta_inte : TransferFcn  Numerator=gyro_bcom  Denominator=gyro_acom
  To Workspace : ToWorkspace  VariableName=phiEst  SampleTime=-1
  To Workspace1 : ToWorkspace  VariableName=thetaEst  SampleTime=-1
  eul2Rot : MATLABFcn  MATLABFcn=quadeul2rotSIMULINK  Output1D=off
  eul2TB : MATLABFcn  MATLABFcn=quadRpqr2euldot  Output1D=off
  Orientation : Outport
  wires:
  stateNon/1 -> Bus Selector1/1, Bus Selector2/1
  IMU/1 -> Bus Selector/1
  Bus Selector1/1 -> Demux3/1  "<eul>"
  Mux/1 -> To Workspace1/1, Scope/1
  Bus Selector2/1 -> Selector2/1  "<euldot>"
  Bus Selector2/2 -> Selector3/1  "<pqr>"
  Mux1/1 -> Scope1/1
  Selector2/1 -> Mux1/1
  Selector3/1 -> Mux1/2
  Mux2/1 -> To Workspace/1, Scope2/1
  Theta_com/1 -> Mux3/2, Mux/2
  Phi_com/1 -> Mux3/1, Mux2/2
  Mux3/1 -> Orientation/1, [eulest]
  Bus Selector/2 -> Multiply/2  "<gyro>"
  eul2TB/1 -> Multiply/1
  Selector4/1 -> Demux1/1
  Gain/1 -> Theta_acc/1, Mux/5
  Gain3/1 -> Phi_acc/1
  Demux1/2 -> Gain3/1
  Demux1/1 -> Gain/1
  Discrete-Time Integrator/1 -> Phi_inte/1
  Demux4/1 -> Discrete-Time Integrator/1
  Discrete-Time Integrator2/1 -> Theta_inte/1
  Demux4/2 -> Discrete-Time Integrator2/1
  Multiply/1 -> Demux4/1
  Demux3/1 -> [Phi_true]  "Phi_true"
  Demux3/2 -> [Theta_true]  "Theta_true"
  Demux3/3 -> [Psi_true]  "Psi_true"
  Demux4/3 -> Terminator1/1
  Bus Selector/1 -> Add1/2  "<acc>"
  Bus Selector1/2 -> [VBdot]  "<vBdot>"
  Constant/1 -> Multiply1/1
  Multiply1/1 -> Add1/1
  Add1/1 -> Selector4/1
  Theta_inte/1 -> [Theta_inte]
  [Theta_inte] -> Add2/2
  Add2/1 -> Theta_com/1
  Add3/1 -> Phi_com/1
  [Psi_true] -> Mux3/3
  [Phi_true] -> Mux2/1
  [Theta_true] -> Mux/1
  [Theta_inte] -> Mux/3
  Phi_inte/1 -> [Phi_inte]
  [Phi_inte] -> Mux2/3
  [Phi_inte] -> Add3/2
  Theta_acc/1 -> [Theta_acc]
  [Theta_acc] -> Add2/1
  [Theta_acc] -> Mux/4
  Phi_acc/1 -> [Phi_acc]
  [Phi_acc] -> Add3/1
  [Phi_acc] -> Mux2/4
  Bus Selector1/3 -> [pdot]  "<pdot>"
  [pdot] -> Multiply2/2
  [VBdot] -> Mux4/2
  Multiply2/1 -> Discrete Derivative/1
  Mux4/1 -> Scope3/1
  Math Function/1 -> Multiply2/1
  Discrete Derivative/1 -> [VBdotest], Mux4/1
  [VBdot] -> Terminator/1
  eul2Rot/1 -> Math Function/1
  [VBdotest] -> Multiply1/2
  [eulest] -> Delay/1
  Delay/1 -> eul2Rot/1, eul2TB/1

== system quadcopterModel/Path Generation/Compute Psi from trajectory ==
  xyz : Inport
  Delay : Delay  DelayLength=1
  Demux : Demux  Outputs=3
  Derivative : Derivative
  Derivative1 : Derivative
  Display : Display
  MATLAB Function : MATLAB Function  TreatAsAtomicUnit=on
  Mux : Mux  Inputs=2
  Mux1 : Mux  Inputs=3
  Scope : Scope
  Terminator : Terminator
  To Workspace5 : ToWorkspace  VariableName=psilem2  SampleTime=-1
  psi : Outport
  wires:
  xyz/1 -> Demux/1
  Demux/1 -> Derivative/1
  Demux/2 -> Derivative1/1
  Demux/3 -> Terminator/1
  MATLAB Function/1(psi) -> To Workspace5/1, psi/1, Mux1/1, Delay/1
  Derivative/1 -> Mux/1
  Derivative1/1 -> Mux/2
  Delay/1 -> MATLAB Function/2(psiOld)
  Mux/1 -> MATLAB Function/1(xydot)
  MATLAB Function/2(psiPure) -> Mux1/2
  Mux1/1 -> Scope/1, Display/1
  MATLAB Function/3(epsi) -> Mux1/3

== system quadcopterModel/Quadcopter/Rotation ==
  pqr : Inport
  U : Inport  Port=2
  param : Inport  Port=3
  3x3 Cross Product : sharedutil/3x3 Cross Product  aMode=aMode
      settings: SourceProductBaseCode=AE
  Add : Sum  Inputs=+--
  Bus Selector : BusSelector  OutputSignals=JMatrix,alphaMatrix
  Multiply : Product  Multiplication=Matrix(*)
  Multiply1 : Product  Multiplication=Matrix(*)
  Multiply3 : Product  Multiplication=Matrix(*)
  Selector : Selector  InputPortWidth=4  IndexOptions=Index vector (dialog)  Indices=[2 3 4]  OutputSizes=1
  inverse J matrix : MATLABFcn  MATLABFcn=inv(u)  Output1D=off
  pqrdot : Outport
  wires:
  U/1 -> Selector/1
  param/1 -> Bus Selector/1
  Bus Selector/1 -> [Jmatrix]  "<JMatrix>"
  Bus Selector/2 -> [alphaMatrix]  "<alphaMatrix>"
  [alphaMatrix] -> Multiply/1
  Multiply/1 -> Add/2
  Selector/1 -> Add/1
  pqr/1 -> 3x3 Cross Product/1, Multiply1/2, Multiply/2
  [Jmatrix] -> Multiply1/1, inverse J matrix/1
  Multiply3/1 -> pqrdot/1
  Add/1 -> Multiply3/2
  inverse J matrix/1 -> Multiply3/1
  Multiply1/1 -> 3x3 Cross Product/2
  3x3 Cross Product/1 -> Add/3

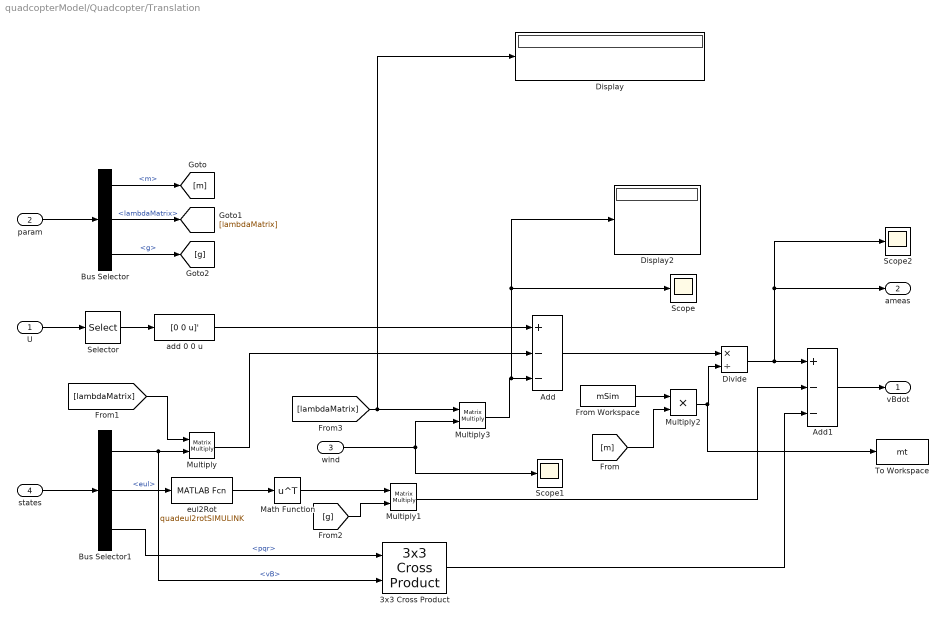
== system quadcopterModel/Quadcopter/Translation ==
  U : Inport
  param : Inport  Port=2
  wind : Inport  Port=3
  states : Inport  Port=4
  3x3 Cross Product : sharedutil/3x3 Cross Product  aMode=aMode
      settings: SourceProductBaseCode=AE
  Add : Sum  Inputs=+--
  Add1 : Sum  Inputs=+--
  Bus Selector : BusSelector  OutputSignals=m,lambdaMatrix,g
  Bus Selector1 : BusSelector  OutputSignals=vB,eul,pqr
  Display : Display
  Display2 : Display
  Divide : Product  Inputs=*/
  From Workspace : FromWorkspace  VariableName=mSim  SampleTime=0
  Math Function : Math  Operator=transpose  SaturateOnIntegerOverflow=on
  Multiply : Product  Multiplication=Matrix(*)
  Multiply1 : Product  Multiplication=Matrix(*)
  Multiply2 : Product
  Multiply3 : Product  Multiplication=Matrix(*)
  Scope : Scope
  Scope1 : Scope
  Scope2 : Scope
  Selector : Selector  InputPortWidth=4  IndexOptions=Index vector (dialog)  Indices=1  OutputSizes=1
  To Workspace : ToWorkspace  VariableName=mt  SampleTime=-1
  add 0 0 u : MATLABFcn  MATLABFcn=[0 0 u]'
  eul2Rot : MATLABFcn  MATLABFcn=quadeul2rotSIMULINK  OutputDimensions=[3 3]  OutputSignalType=real  Output1D=off
  vBdot : Outport
  ameas : Outport  Port=2
  wires:
  U/1 -> Selector/1
  Selector/1 -> add 0 0 u/1
  param/1 -> Bus Selector/1
  Bus Selector/1 -> [m]  "<m>"
  Bus Selector/2 -> [lambdaMatrix]  "<lambdaMatrix>"
  Bus Selector/3 -> [g]  "<g>"
  add 0 0 u/1 -> Add/1
  Add/1 -> Divide/1
  states/1 -> Bus Selector1/1
  Bus Selector1/1 -> 3x3 Cross Product/2, Multiply/2  "<vB>"
  [lambdaMatrix] -> Multiply/1
  Multiply/1 -> Add/2
  Bus Selector1/2 -> eul2Rot/1  "<eul>"
  [g] -> Multiply1/2
  Divide/1 -> Scope2/1, ameas/1, Add1/1
  Multiply1/1 -> Add1/2
  Add1/1 -> vBdot/1
  Math Function/1 -> Multiply1/1
  [lambdaMatrix] -> Display/1, Multiply3/1
  Multiply3/1 -> Display2/1, Scope/1, Add/3
  Bus Selector1/3 -> 3x3 Cross Product/1  "<pqr>"
  3x3 Cross Product/1 -> Add1/3
  eul2Rot/1 -> Math Function/1
  wind/1 -> Multiply3/2, Scope1/1
  From Workspace/1 -> Multiply2/1
  Multiply2/1 -> To Workspace/1, Divide/2
  [m] -> Multiply2/2

== system quadcopterModel/Quadcopter/addNoiseToIMU ==
  a_noNoise : Inport
  gyr_noNoise : Inport  Port=2
  Add : Sum
  Add1 : Sum
  Demux : Demux  Outputs=3
  From Workspace : FromWorkspace  VariableName=eacc  SampleTime=0
  From Workspace1 : FromWorkspace  VariableName=egyro  SampleTime=0
  Gain : Gain  Gain=gainAcc
  Gain1 : Gain  Gain=gainGyro
  Mux : Mux  Inputs=3
  Transfer Fcn : TransferFcn  Numerator=bgyro  Denominator=agyro
  Transfer Fcn1 : TransferFcn  Numerator=bgyro  Denominator=agyro
  Transfer Fcn2 : TransferFcn  Numerator=bgyro  Denominator=agyro
  acc : Outport
  gyro : Outport  Port=2
  gyro0 : Outport  Port=3
  wires:
  Add1/1 -> gyro/1  "gyro"
  From Workspace/1 -> Gain/1
  a_noNoise/1 -> Add/2
  gyr_noNoise/1 -> gyro0/1, Add1/2
  Add/1 -> acc/1  "acc"
  From Workspace1/1 -> Demux/1
  Demux/1 -> Transfer Fcn/1
  Demux/2 -> Transfer Fcn1/1
  Demux/3 -> Transfer Fcn2/1
  Transfer Fcn/1 -> Mux/1
  Transfer Fcn1/1 -> Mux/2
  Transfer Fcn2/1 -> Mux/3
  Mux/1 -> Gain1/1
  Gain/1 -> Add/1
  Gain1/1 -> Add1/1

== system quadcopterModel/Quadcopter1/Rotation ==
  pqr : Inport
  U : Inport  Port=2
  param : Inport  Port=3
  3x3 Cross Product : sharedutil/3x3 Cross Product  aMode=aMode
      settings: SourceProductBaseCode=AE
  Add : Sum  Inputs=+--
  Bus Selector : BusSelector  OutputSignals=JMatrix,alphaMatrix
  Multiply : Product  Multiplication=Matrix(*)
  Multiply1 : Product  Multiplication=Matrix(*)
  Multiply3 : Product  Multiplication=Matrix(*)
  Selector : Selector  InputPortWidth=4  IndexOptions=Index vector (dialog)  Indices=[2 3 4]  OutputSizes=1
  inverse J matrix : MATLABFcn  MATLABFcn=inv(u)  Output1D=off
  pqrdot : Outport
  wires:
  3x3 Cross Product/1 -> Add/3
  Multiply1/1 -> 3x3 Cross Product/2
  inverse J matrix/1 -> Multiply3/1
  Add/1 -> Multiply3/2
  Multiply3/1 -> pqrdot/1
  [Jmatrix] -> inverse J matrix/1, Multiply1/1
  pqr/1 -> Multiply/2, Multiply1/2, 3x3 Cross Product/1
  Selector/1 -> Add/1
  Multiply/1 -> Add/2
  [alphaMatrix] -> Multiply/1
  Bus Selector/2 -> [alphaMatrix]  "<alphaMatrix>"
  Bus Selector/1 -> [Jmatrix]  "<JMatrix>"
  param/1 -> Bus Selector/1
  U/1 -> Selector/1
